simulink model "ABS_ameliore"  (R2022b)
settings: Solver=VariableStepAuto  StartTime=0.0  StopTime=15  RelTol=1e-3
values from neighbouring files (symbols this model uses):
  gp = 9.81    [ABS_config.m]
  J = 0.5    [ABS_config.m]
  m = 1000    [ABS_config.m]
  rR = 0.3    [ABS_config.m]
  V0 = 27.77    [ABS_config.m]
  w0 = V0/rR    (= 92.5666666667)    [ABS_config.m]
libraries: simulink x2, slpidlib x2
settings Model: Creator=elmeh  LastModifiedBy=Youssef ABLALI
settings SolverCC: ZeroCrossAlgorithm=Adaptive
settings DebuggingCC: IgnoredZcDiagnostic=none

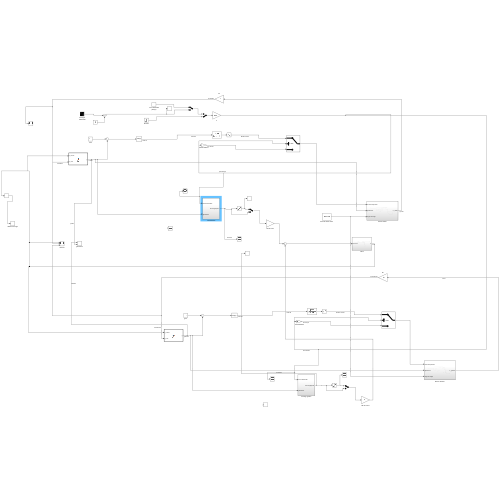
[thumbnail: Simulink's stored preview of the top-level diagram]
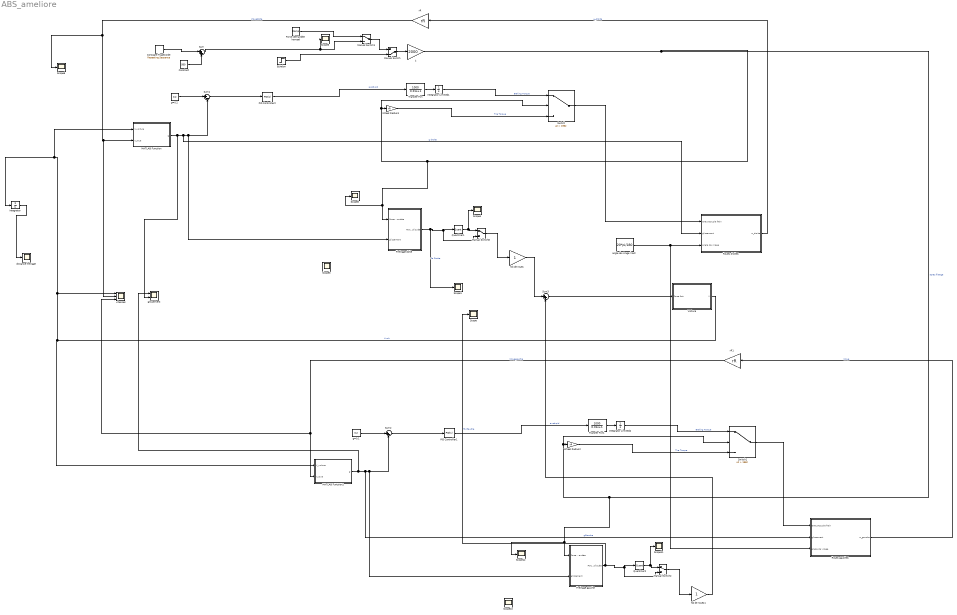
== system ABS_ameliore ==
  Consigne Trapézoide : simulink/Sources/Repeating Sequence  rep_seq_t=[0 0.1 0.2 0.3 0.4 0.5]  rep_seq_y=[0 1000 1000 1000 0 0]
  Constant : Constant  Value=500
  Echelon : Step  SampleTime=0
  Force demandée (rampe) : simulink/Sources/Ramp  slope=1  start=0  InitialOutput=0
  Freinage doite : Subsystem
  Freinage gauche : Subsystem
  Integrator : Integrator  LimitOutput=on  LowerSaturationLimit=0
  Integrator Limited1 : Integrator  LimitOutput=on  UpperSaturationLimit=1500  LowerSaturationLimit=0
  Integrator Limited2 : Integrator  LimitOutput=on  UpperSaturationLimit=1500  LowerSaturationLimit=0
  MATLAB Function : MATLAB Function  TreatAsAtomicUnit=on
  MATLAB Function1 : MATLAB Function  TreatAsAtomicUnit=on
  Manual Switch : ManualSwitch  CurrentSetting=0
  Manual Switch1 : ManualSwitch
  Manual Switch2 : ManualSwitch
  Manual Switch8 : ManualSwitch
  Nb de roues : Gain
  Nb de roues1 : Gain
  PID Controller1 : slpidlib/PID Controller  Controller=PID  Form=Parallel  TimeDomain=Continuous-time  UseExternalTs=off  SampleTime=-1  IntegratorMethod=Forward Euler  FilterMethod=Forward Euler  ControllerParametersSource=internal  P=50  I=1  UseKiTs=off  D=5  N=100  UseFilter=on  TunerSelectOption=Transfer Function Based (PID Tuner App)  InitialConditionSource=internal  InitialConditionForIntegrator=0  InitialConditionForFilter=0  DifferentiatorICPrevScaledInput=0  ExternalReset=none  TrackingMode=off  Kt=1  LimitOutput=off  SatLimitsSource=internal  UpperSaturationLimit=inf  LowerSaturationLimit=-inf  LinearizeAsGain=on  AntiWindupMode=none  Kb=1  LimitIntegrator=off  UpperIntegratorSaturationLimit=inf  LowerIntegratorSaturationLimit=-inf  POutMin=[]  POutMax=[]  IOutMin=[]  IOutMax=[]  DOutMin=[]  DOutMax=[]  NOutMin=[]  NOutMax=[]  SumOutMin=[]  SumOutMax=[]  SaturationOutMin=[]  SaturationOutMax=[]  PParamMin=[]  PParamMax=[]  IParamMin=[]  IParamMax=[]  DParamMin=[]  DParamMax=[]  NParamMin=[]  NParamMax=[]  KbParamMin=[]  KbParamMax=[]  KtParamMin=[]  KtParamMax=[]  KbOutMin=[]  KbOutMax=[]  KtOutMin=[]  KtOutMax=[]  IntegratorOutMin=[]  IntegratorOutMax=[]  FilterOutMin=[]  FilterOutMax=[]  SumI1OutMin=[]  SumI1OutMax=[]  SumI2OutMin=[]  SumI2OutMax=[]  SumI3OutMin=[]  SumI3OutMax=[]  SumI4OutMin=[]  SumI4OutMax=[]  SumDOutMin=[]  SumDOutMax=[]  DifferentiatorOutMin=[]  DifferentiatorOutMax=[]  FilterDiffOutCoefMin=[]  FilterDiffOutCoefMax=[]  ReciprocalOutMin=[]  ReciprocalOutMax=[]  SumDenOutMin=[]  SumDenOutMax=[]  SumNumOutMin=[]  SumNumOutMax=[]  DivideOutMin=[]  DivideOutMax=[]  UdiffTsProdOutMin=[]  UdiffTsProdOutMax=[]  NTsProdOutMin=[]  NTsProdOutMax=[]  UintegralTsProdOutMin=[]  UintegralTsProdOutMax=[]  UngainTsProdOutMin=[]  UngainTsProdOutMax=[]  ClampingZeroOutDataTypeStr=Inherit: Inherit via back propagation  ClampingZeroOutMin=[]  ClampingZeroOutMax=[]  FilterDenConstantOutDataTypeStr=Inherit: Inherit via back propagation  FilterDenConstantOutMin=[]  FilterDenConstantOutMax=[]  PCopyOutDataTypeStr=Inherit: Inherit via back propagation  PCopyOutMin=[]  PCopyOutMax=[]  NCopyOutDataTypeStr=Inherit: Inherit via back propagation  NCopyOutMin=[]  NCopyOutMax=[]  IntegratorContinuousStateAttributes=''  IntegratorStateMustResolveToSignalObject=off  IntegratorRTWStateStorageClass=Auto  FilterContinuousStateAttributes=''  FilterStateMustResolveToSignalObject=off  FilterRTWStateStorageClass=Auto  ParallelPVariant=InternalParameters  IdealPVariant=Disabled  IVariant=InternalParameters  DVariant=InternalParameters  IntegratorVariant=Continuous  SatVariant=Disabled  AWVariant=Passthrough  PCopyVariant=Disabled  TRVariant=Disabled  FdbkBlocksVariant=Forward  IdealPFdbkVariant=Disabled  SatFdbkVariant=Disabled  DerivativeFilterVariant=ContFilter  NVariant=InternalParameters  NCopyVariant=Disabled  FilterICVariant=InternalICsFilter  IntegratorICVariant=InternalICs  ExternalResetVariant=Disabled  TRSumVariant=Passthrough  SumFdbkVariant=Disabled  SumVariant=Sum_PID  TsampFilterVariant=InternalTs  TsampNgainVariant=Passthrough  TsampIntegralVariant=Passthrough  ExternalSaturationOutDataTypeStr=Inherit: Same as second input
  PID Controller2 : slpidlib/PID Controller  Controller=PID  Form=Parallel  TimeDomain=Continuous-time  UseExternalTs=off  SampleTime=-1  IntegratorMethod=Forward Euler  FilterMethod=Forward Euler  ControllerParametersSource=internal  P=50  I=1  UseKiTs=off  D=5  N=100  UseFilter=on  TunerSelectOption=Transfer Function Based (PID Tuner App)  InitialConditionSource=internal  InitialConditionForIntegrator=0  InitialConditionForFilter=0  DifferentiatorICPrevScaledInput=0  ExternalReset=none  TrackingMode=off  Kt=1  LimitOutput=off  SatLimitsSource=internal  UpperSaturationLimit=inf  LowerSaturationLimit=-inf  LinearizeAsGain=on  AntiWindupMode=none  Kb=1  LimitIntegrator=off  UpperIntegratorSaturationLimit=inf  LowerIntegratorSaturationLimit=-inf  POutMin=[]  POutMax=[]  IOutMin=[]  IOutMax=[]  DOutMin=[]  DOutMax=[]  NOutMin=[]  NOutMax=[]  SumOutMin=[]  SumOutMax=[]  SaturationOutMin=[]  SaturationOutMax=[]  PParamMin=[]  PParamMax=[]  IParamMin=[]  IParamMax=[]  DParamMin=[]  DParamMax=[]  NParamMin=[]  NParamMax=[]  KbParamMin=[]  KbParamMax=[]  KtParamMin=[]  KtParamMax=[]  KbOutMin=[]  KbOutMax=[]  KtOutMin=[]  KtOutMax=[]  IntegratorOutMin=[]  IntegratorOutMax=[]  FilterOutMin=[]  FilterOutMax=[]  SumI1OutMin=[]  SumI1OutMax=[]  SumI2OutMin=[]  SumI2OutMax=[]  SumI3OutMin=[]  SumI3OutMax=[]  SumI4OutMin=[]  SumI4OutMax=[]  SumDOutMin=[]  SumDOutMax=[]  DifferentiatorOutMin=[]  DifferentiatorOutMax=[]  FilterDiffOutCoefMin=[]  FilterDiffOutCoefMax=[]  ReciprocalOutMin=[]  ReciprocalOutMax=[]  SumDenOutMin=[]  SumDenOutMax=[]  SumNumOutMin=[]  SumNumOutMax=[]  DivideOutMin=[]  DivideOutMax=[]  UdiffTsProdOutMin=[]  UdiffTsProdOutMax=[]  NTsProdOutMin=[]  NTsProdOutMax=[]  UintegralTsProdOutMin=[]  UintegralTsProdOutMax=[]  UngainTsProdOutMin=[]  UngainTsProdOutMax=[]  ClampingZeroOutDataTypeStr=Inherit: Inherit via back propagation  ClampingZeroOutMin=[]  ClampingZeroOutMax=[]  FilterDenConstantOutDataTypeStr=Inherit: Inherit via back propagation  FilterDenConstantOutMin=[]  FilterDenConstantOutMax=[]  PCopyOutDataTypeStr=Inherit: Inherit via back propagation  PCopyOutMin=[]  PCopyOutMax=[]  NCopyOutDataTypeStr=Inherit: Inherit via back propagation  NCopyOutMin=[]  NCopyOutMax=[]  IntegratorContinuousStateAttributes=''  IntegratorStateMustResolveToSignalObject=off  IntegratorRTWStateStorageClass=Auto  FilterContinuousStateAttributes=''  FilterStateMustResolveToSignalObject=off  FilterRTWStateStorageClass=Auto  ParallelPVariant=InternalParameters  IdealPVariant=Disabled  IVariant=InternalParameters  DVariant=InternalParameters  IntegratorVariant=Continuous  SatVariant=Disabled  AWVariant=Passthrough  PCopyVariant=Disabled  TRVariant=Disabled  FdbkBlocksVariant=Forward  IdealPFdbkVariant=Disabled  SatFdbkVariant=Disabled  DerivativeFilterVariant=ContFilter  NVariant=InternalParameters  NCopyVariant=Disabled  FilterICVariant=InternalICsFilter  IntegratorICVariant=InternalICs  ExternalResetVariant=Disabled  TRSumVariant=Passthrough  SumFdbkVariant=Disabled  SumVariant=Sum_PID  TsampFilterVariant=InternalTs  TsampNgainVariant=Passthrough  TsampIntegralVariant=Passthrough  ExternalSaturationOutDataTypeStr=Inherit: Same as second input
  Quantizer1 : Quantizer  QuantizationInterval=400
  Quantizer2 : Quantizer  QuantizationInterval=400
  Roues droites : Subsystem
  Roues gauches : Subsystem
  Scope{,1,3..6,8,10..12} (10 alike) : Scope
  Sum : Sum  Inputs=|++
  Sum1 : Sum  Inputs=|+-
  Sum2 : Sum  Inputs=|+-
  Sum3 : Sum  Inputs=|++
  Switch : Switch  Criteria=u2 > Threshold  Threshold=1962  SaturateOnIntegerOverflow=off  InputSameDT=off
  Switch1 : Switch  Criteria=u2 > Threshold  Threshold=1962  SaturateOnIntegerOverflow=off  InputSameDT=off
  Transfer Fcn : TransferFcn  Numerator=[1000]  Denominator=[0.01 1]
  Transfer Fcn1 : TransferFcn  Numerator=[1000]  Denominator=[0.01 1]
  Voiture : Subsystem
  Wheel Radius1 : Gain  Gain=rR
  Wheel Radius2 : Gain  Gain=rR
  angle de virage (rad) : Constant  Value=20*pi/180
  distance freinage : Scope
  g=0.1 : Constant  Value=0.2
  g=0.2 : Constant  Value=0.2
  glissement : Scope  NumInputPorts=2
  k : Gain  Gain=2000
  rR : Gain  Gain=rR
  rR1 : Gain  Gain=rR
  vitesses : Scope  NumInputPorts=3
  wires:
  Force demandée (rampe)/1 -> Manual Switch1/1
  Echelon/1 -> Manual Switch/2
  Manual Switch1/1 -> Manual Switch/1
  Sum/1 -> Scope5/1, Manual Switch1/2
  Sum3/1 -> Voiture/1(Force frot)
  Manual Switch/1 -> k/1
  Roues droites/1(ω_droite) -> rR/1  "ω_droite"
  rR/1 -> vitesses/2, MATLAB Function/2(V_roue), Scope6/1  "Vrouedoite"
  Voiture/1("V ") -> MATLAB Function1/1(V_voiture), Integrator/1, MATLAB Function/1(V_voiture), vitesses/1  "Vvoit"
  Integrator/1 -> distance freinage/1
  Freinage doite/1("Force Appliquée ") -> Scope1/1, Manual Switch8/2, Quantizer1/1  "Fa Droite"
  Quantizer1/1 -> Scope4/1, Manual Switch8/1
  Manual Switch8/1 -> Nb de roues/1
  Consigne Trapézoide/1 -> Sum/1
  Constant/1 -> Sum/2
  g=0.2/1 -> Sum1/1
  MATLAB Function/1(g) -> Roues droites/2(glissement), Freinage doite/2("glissement "), Sum1/2, glissement/2  "g droite"
  Sum1/1 -> PID Controller2/1
  Wheel Radius1/1 -> Switch/3  "Tire Torque"
  Switch/1 -> Roues droites/1(erreur/Couple frein)
  Transfer Fcn/1 -> Integrator Limited1/1
  Integrator Limited1/1 -> Switch/1  "Braking Torque"
  PID Controller2/1 -> Transfer Fcn/1  "avatt pid"
  Roues gauches/1(ω_gauche) -> rR1/1  "Vroue"
  PID Controller1/1 -> Transfer Fcn1/1  "avatt pid"
  Transfer Fcn1/1 -> Integrator Limited2/1
  g=0.1/1 -> Sum2/1
  Switch1/1 -> Roues gauches/1(erreur/Couple frein)
  Wheel Radius2/1 -> Switch1/3  "Tire Torque"
  MATLAB Function1/1(g) -> glissement/1, Roues gauches/2(glissement), Freinage gauche/2("glissement "), Sum2/2  "gGauche"
  Sum2/1 -> PID Controller1/1
  Manual Switch2/1 -> Nb de roues1/1
  Integrator Limited2/1 -> Switch1/1  "Braking Torque"
  Quantizer2/1 -> Scope11/1, Manual Switch2/1
  k/1 -> Switch1/2, Wheel Radius2/1, Scope12/1, Freinage gauche/1(Force demandée), Switch/2, Wheel Radius1/1, Scope8/1, Freinage doite/1(Force demandée)  "apres filtrage"
  Freinage gauche/1("Force Appliquée ") -> Scope/1, Manual Switch2/2, Quantizer2/1  "Fa Gauche"
  angle de virage (rad)/1 -> Roues gauches/3(angle de virage), Roues droites/3(angle de virage)
  rR1/1 -> vitesses/3, MATLAB Function1/2(V_roue)  "Vrouegauche"
  Nb de roues/1 -> Sum3/1
  Nb de roues1/1 -> Sum3/2

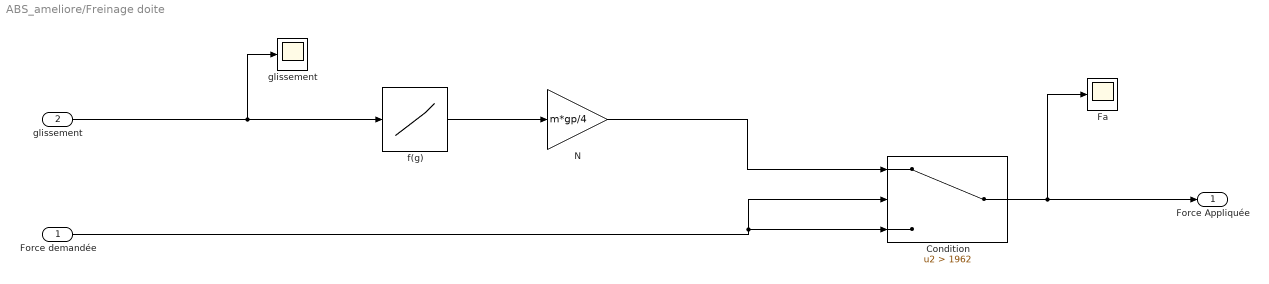
== system ABS_ameliore/Freinage doite ==
  Force demandée : Inport
  "glissement " : Inport  Port=2
  "Condition " : Switch  Criteria=u2 > Threshold  Threshold=1962  SaturateOnIntegerOverflow=off  InputSameDT=off
  "Fa " : Scope
  N : Gain  Gain=m*gp/4
  f(g) : Lookup_n-D  NumberOfTableDimensions=1  BreakpointsForDimension1=[0,0.1,0.2,0.3,0.4,0.5,0.6,0.7,0.8,0.9,1.0]  Table=[0.0,0.85,0.95,0.78,0.73,0.7,0.68,0.66,0.64,0.62,0.61]  InternalRulePriority=Speed  RndMeth=Simplest
  glissement : Scope
  "Force Appliquée " : Outport  VectorParamsAs1DForOutWhenUnconnected=off
  wires:
  f(g)/1 -> N/1
  Force demandée/1 -> "Condition "/3, "Condition "/2
  "glissement "/1 -> f(g)/1, glissement/1
  "Condition "/1 -> "Force Appliquée "/1, "Fa "/1
  N/1 -> "Condition "/1

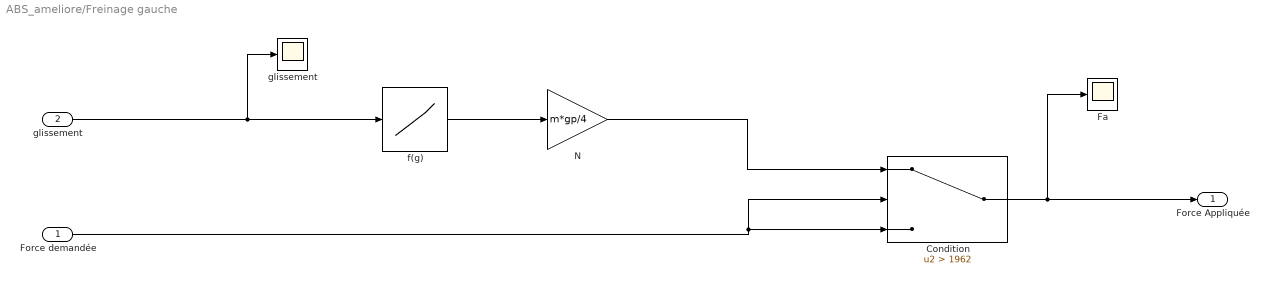
== system ABS_ameliore/Freinage gauche ==
  Force demandée : Inport
  "glissement " : Inport  Port=2
  "Condition " : Switch  Criteria=u2 > Threshold  Threshold=1962  SaturateOnIntegerOverflow=off  InputSameDT=off
  "Fa " : Scope
  N : Gain  Gain=m*gp/4
  f(g) : Lookup_n-D  NumberOfTableDimensions=1  BreakpointsForDimension1=[0,0.1,0.2,0.3,0.4,0.5,0.6,0.7,0.8,0.9,1.0]  Table=[0.0,0.85,0.95,0.78,0.73,0.7,0.68,0.66,0.64,0.62,0.61]  InternalRulePriority=Speed  RndMeth=Simplest
  glissement : Scope
  "Force Appliquée " : Outport  VectorParamsAs1DForOutWhenUnconnected=off
  wires:
  f(g)/1 -> N/1
  Force demandée/1 -> "Condition "/3, "Condition "/2
  "glissement "/1 -> f(g)/1, glissement/1
  "Condition "/1 -> "Force Appliquée "/1, "Fa "/1
  N/1 -> "Condition "/1

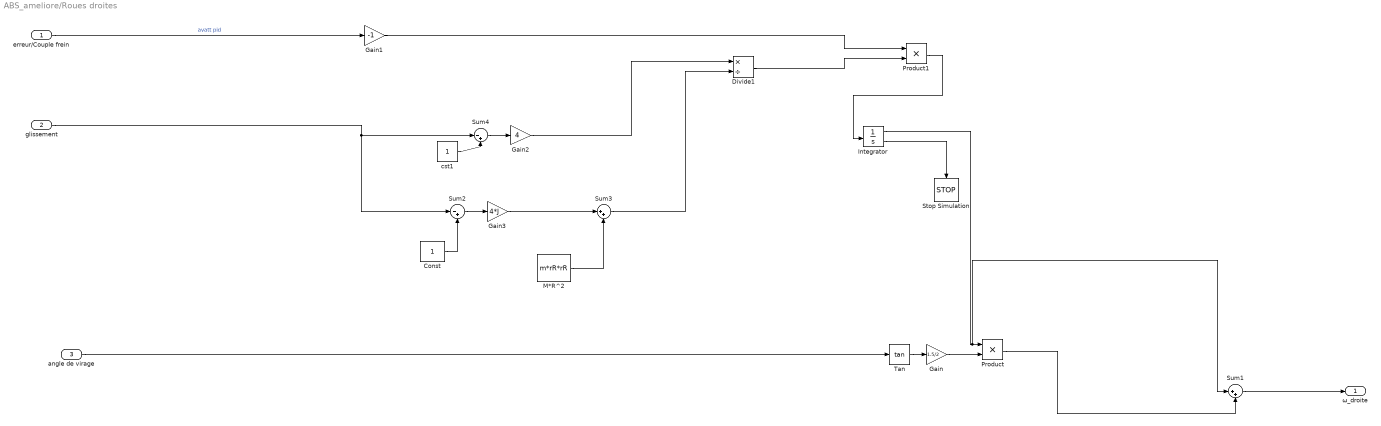
== system ABS_ameliore/Roues droites ==
  erreur/Couple frein : Inport
  glissement : Inport  Port=2
  angle de virage : Inport  Port=3
  Const : Constant
  Divide1 : Product  Inputs=*/
  Gain : Gain  Gain=1.5/2
  Gain1 : Gain  Gain=-1
  Gain2 : Gain  Gain=4
  Gain3 : Gain  Gain=4*J
  Integrator : Integrator  InitialCondition=w0  LimitOutput=on  LowerSaturationLimit=0  ShowSaturationPort=on
  M*R^2 : Constant  Value=m*rR*rR
  Product : Product
  Product1 : Product
  Stop Simulation : Stop
  Sum1 : Sum  Inputs=|++
  Sum2 : Sum  Inputs=|-+
  Sum3 : Sum  Inputs=|++
  Sum4 : Sum  Inputs=|-+
  Tan : Trigonometry  Operator=tan
  cst1 : Constant
  ω_droite : Outport
  wires:
  Integrator/2 -> Stop Simulation/1
  Product1/1 -> Integrator/1
  glissement/1 -> Sum2/1, Sum4/1
  Const/1 -> Sum2/2
  M*R^2/1 -> Sum3/2
  Sum3/1 -> Divide1/2
  Gain2/1 -> Divide1/1
  Gain1/1 -> Product1/1
  Sum2/1 -> Gain3/1
  Sum4/1 -> Gain2/1
  Divide1/1 -> Product1/2
  Gain3/1 -> Sum3/1
  cst1/1 -> Sum4/2
  Integrator/1 -> Sum1/1, Product/1
  erreur/Couple frein/1 -> Gain1/1  "avatt pid"
  Gain/1 -> Product/2
  Tan/1 -> Gain/1
  Product/1 -> Sum1/2
  angle de virage/1 -> Tan/1
  Sum1/1 -> ω_droite/1

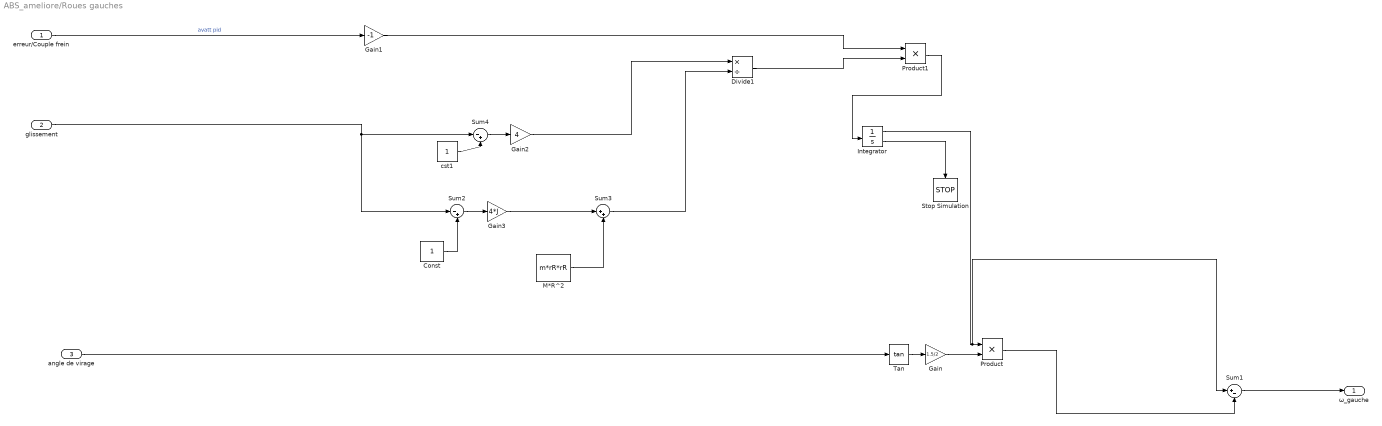
== system ABS_ameliore/Roues gauches ==
  erreur/Couple frein : Inport
  glissement : Inport  Port=2
  angle de virage : Inport  Port=3
  Const : Constant
  Divide1 : Product  Inputs=*/
  Gain : Gain  Gain=1.5/2
  Gain1 : Gain  Gain=-1
  Gain2 : Gain  Gain=4
  Gain3 : Gain  Gain=4*J
  Integrator : Integrator  InitialCondition=w0  LimitOutput=on  LowerSaturationLimit=0  ShowSaturationPort=on
  M*R^2 : Constant  Value=m*rR*rR
  Product : Product
  Product1 : Product
  Stop Simulation : Stop
  Sum1 : Sum  Inputs=|+-
  Sum2 : Sum  Inputs=|-+
  Sum3 : Sum  Inputs=|++
  Sum4 : Sum  Inputs=|-+
  Tan : Trigonometry  Operator=tan
  cst1 : Constant
  ω_gauche : Outport
  wires:
  Integrator/2 -> Stop Simulation/1
  Product1/1 -> Integrator/1
  glissement/1 -> Sum2/1, Sum4/1
  Const/1 -> Sum2/2
  M*R^2/1 -> Sum3/2
  Sum3/1 -> Divide1/2
  Gain2/1 -> Divide1/1
  Gain1/1 -> Product1/1
  Sum2/1 -> Gain3/1
  Sum4/1 -> Gain2/1
  Divide1/1 -> Product1/2
  Gain3/1 -> Sum3/1
  cst1/1 -> Sum4/2
  Integrator/1 -> Sum1/1, Product/1
  erreur/Couple frein/1 -> Gain1/1  "avatt pid"
  Gain/1 -> Product/2
  Tan/1 -> Gain/1
  Product/1 -> Sum1/2
  angle de virage/1 -> Tan/1
  Sum1/1 -> ω_gauche/1

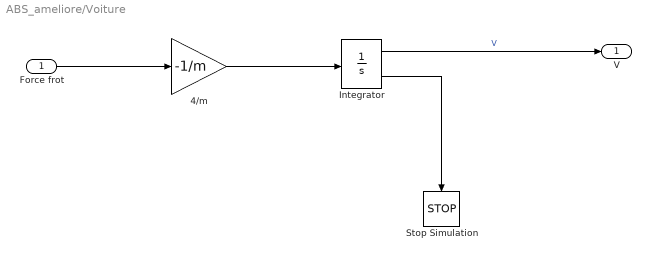
== system ABS_ameliore/Voiture ==
  Force frot : Inport
  4/m : Gain  Gain=-1/m
  Integrator : Integrator  InitialCondition=V0  LimitOutput=on  LowerSaturationLimit=0  ShowSaturationPort=on
  Stop Simulation : Stop
  "V " : Outport
  wires:
  Force frot/1 -> 4/m/1
  4/m/1 -> Integrator/1
  Integrator/1 -> "V "/1  "V"
  Integrator/2 -> Stop Simulation/1

== matlab function ABS_ameliore/MATLAB Function ==
  data: V_voiture input; V_roue input; g output
function g = fcn(V_voiture,V_roue)

g = (V_voiture - V_roue)/V_voiture;

== matlab function ABS_ameliore/MATLAB Function1 ==
  data: V_voiture input; V_roue input; g output
function g = fcn(V_voiture,V_roue)

g = (V_voiture - V_roue)/V_voiture;
